simulink model "BLOC_Differential"  (R2016a)
settings: Solver=VariableStepAuto  StartTime=0.0  StopTime=10.0  RelTol=1e-3
undefined symbols (not defined in the file): hev_dt, ra_differential_ratio, ra_transmission_efficiency
settings Model: Creator=Florent  LastModifiedBy=Florent

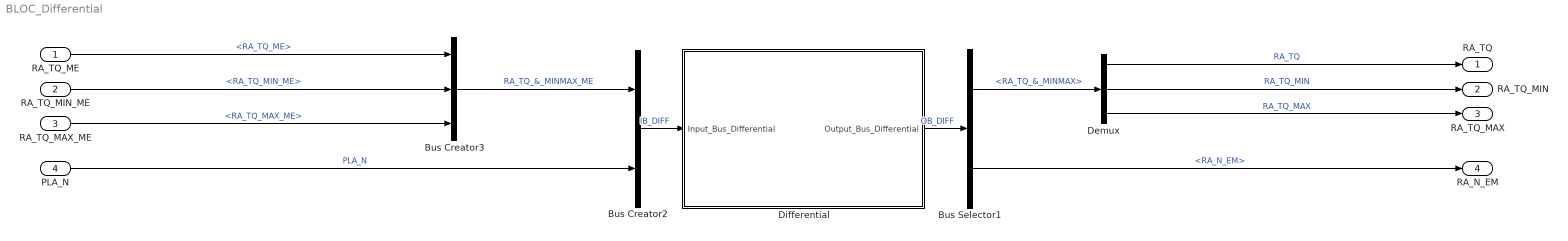
== system BLOC_Differential ==
  RA_TQ_ME : Inport
  RA_TQ_MIN_ME : Inport  Port=2
  RA_TQ_MAX_ME : Inport  Port=3
  PLA_N : Inport  Port=4
  Bus Creator2 : BusCreator  Inputs=2
  Bus Creator3 : BusCreator  Inputs=3
  Bus Selector1 : BusSelector  OutputSignals=RA_TQ_&_MINMAX,RA_N_EM
  Demux : Demux  Outputs=3
  Differential : Subsystem  TreatAsAtomicUnit=on  SystemSampleTime=hev_dt
  RA_TQ : Outport
  RA_TQ_MIN : Outport  Port=2
  RA_TQ_MAX : Outport  Port=3
  RA_N_EM : Outport  Port=4
  wires:
  Bus Creator3/1 -> Bus Creator2/1  "RA_TQ_&_MINMAX_ME"
  Demux/1 -> RA_TQ/1  "RA_TQ"
  Demux/3 -> RA_TQ_MAX/1  "RA_TQ_MAX"
  Demux/2 -> RA_TQ_MIN/1  "RA_TQ_MIN"
  PLA_N/1 -> Bus Creator2/2  "PLA_N"
  Differential/1(Output_Bus_Differential) -> Bus Selector1/1  "OB_DIFF"
  Bus Selector1/2 -> RA_N_EM/1  "<RA_N_EM>"
  Bus Selector1/1 -> Demux/1  "<RA_TQ_&_MINMAX>"
  Bus Creator2/1 -> Differential/1("Input_Bus_Differential ")  "IB_DIFF"
  RA_TQ_ME/1 -> Bus Creator3/1  "<RA_TQ_ME>"
  RA_TQ_MIN_ME/1 -> Bus Creator3/2  "<RA_TQ_MIN_ME>"
  RA_TQ_MAX_ME/1 -> Bus Creator3/3  "<RA_TQ_MAX_ME>"

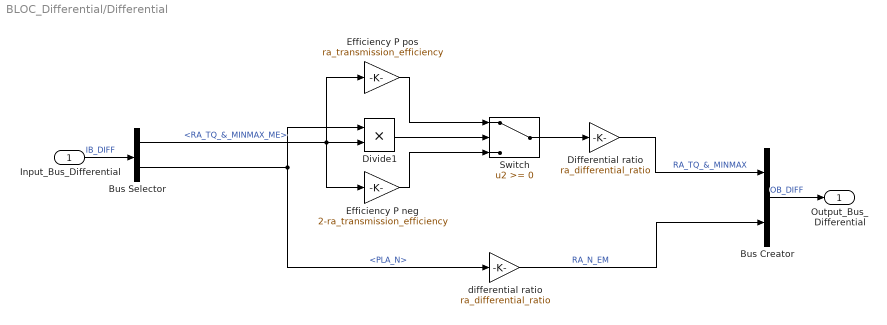
== system BLOC_Differential/Differential ==
  "Input_Bus_Differential " : Inport
  Bus Creator : BusCreator  Inputs=2
  Bus Selector : BusSelector  OutputSignals=RA_TQ_&_MINMAX_ME,PLA_N
  Differential ratio : Gain  Gain=ra_differential_ratio  SampleTime=hev_dt
  Divide1 : Product  SampleTime=hev_dt
  Efficiency P neg : Gain  Gain=2-ra_transmission_efficiency  SampleTime=hev_dt
  Efficiency P pos : Gain  Gain=ra_transmission_efficiency  SampleTime=hev_dt
  Switch : Switch  SampleTime=hev_dt
  differential ratio : Gain  Gain=ra_differential_ratio  SampleTime=hev_dt
  Output_Bus_Differential : Outport
  wires:
  Efficiency P pos/1 -> Switch/1
  Efficiency P neg/1 -> Switch/3
  Divide1/1 -> Switch/2
  Switch/1 -> Differential ratio/1
  Differential ratio/1 -> Bus Creator/1  "RA_TQ_&_MINMAX"
  differential ratio/1 -> Bus Creator/2  "RA_N_EM"
  Bus Creator/1 -> Output_Bus_Differential/1  "OB_DIFF"
  "Input_Bus_Differential "/1 -> Bus Selector/1  "IB_DIFF"
  Bus Selector/2 -> differential ratio/1, Divide1/1  "<PLA_N>"
  Bus Selector/1 -> Efficiency P neg/1, Divide1/2, Efficiency P pos/1  "<RA_TQ_&_MINMAX_ME>"
